simulink model "beam_model"  (R2025b)
settings: Solver=VariableStepAuto  StartTime=0.0  StopTime=10.0  RelTol=1e-3
settings Model: Creator=hm-egod12az  LastModifiedBy=hm-egod12az

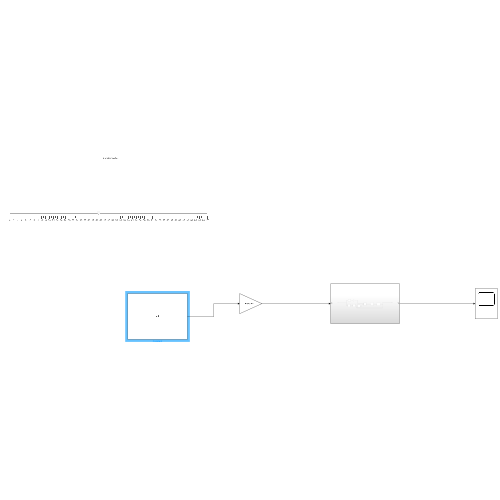
[thumbnail: Simulink's stored preview of the top-level diagram]
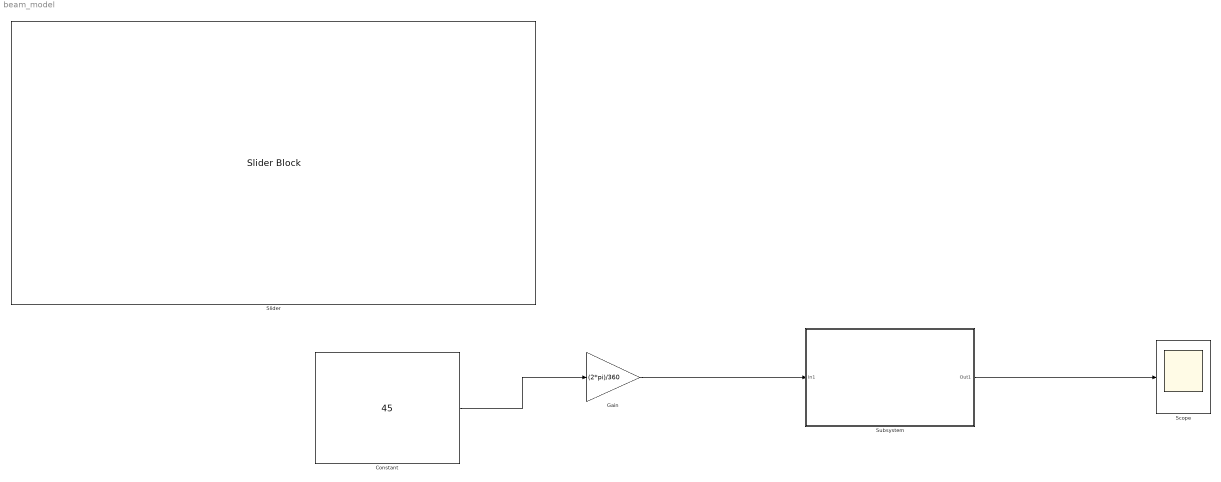
== system beam_model ==
  Constant : Constant  Value=45
  Gain : Gain  Gain=(2*pi)/360
  Scope : Scope
      settings: ActiveDisplayYMinimum=-390.19036069350165  ActiveDisplayYMaximum=43.354484521500176
  Slider : SliderBlock
  Subsystem : Subsystem
  wires:
  Constant/1 -> Gain/1
  Subsystem/1(Out1) -> Scope/1
  Gain/1 -> Subsystem/1(In1)

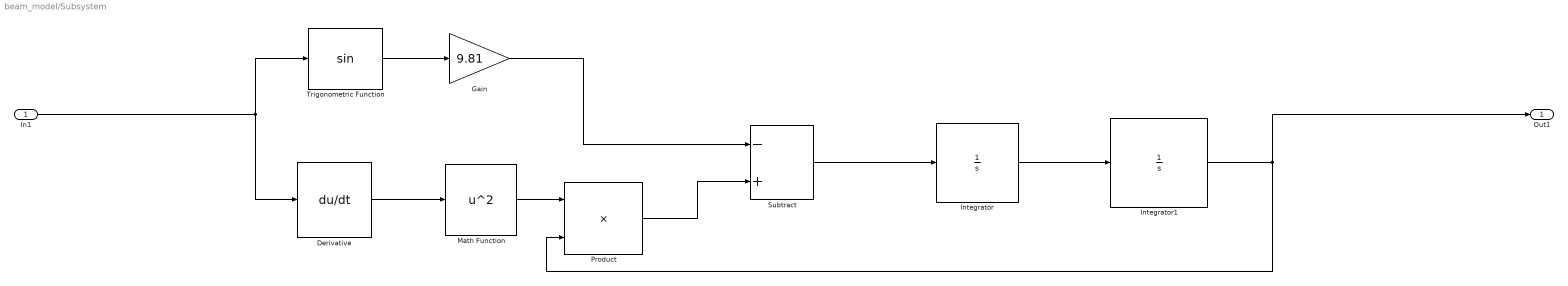
== system beam_model/Subsystem ==
  In1 : Inport
  Derivative : Derivative
  Gain : Gain  Gain=9.81
  Integrator : Integrator
  Integrator1 : Integrator
  Math Function : Math  Operator=square
  Product : Product
  Subtract : Sum  Inputs=-+
  Trigonometric Function : Trigonometry
  Out1 : Outport
  wires:
  Derivative/1 -> Math Function/1
  Integrator1/1 -> Out1/1, Product/2
  Math Function/1 -> Product/1
  In1/1 -> Derivative/1, Trigonometric Function/1
  Product/1 -> Subtract/2
  Gain/1 -> Subtract/1
  Subtract/1 -> Integrator/1
  Trigonometric Function/1 -> Gain/1
  Integrator/1 -> Integrator1/1
